simulink model "TRAS_pitch_model"  (Simulink 8.3)
settings: Solver=ode5  StartTime=0.0  StopTime=75  FixedStep=.01  RelTol=1e-3
PreLoadFcn:
  | load tras_char
undefined symbols (not defined in the file): control_p, force_p, rpm_p
settings Model: Creator=inteco  LastModifiedBy=inteco
settings DataIOCC: SignalLoggingName=sigsOut
settings OptimizationCC: ExpressionDepthLimit=2147483647
settings DebuggingCC: SaveWithParameterizedLinksMsg=none  SignalResolutionControl=TryResolveAllWithWarning  SolverPrmCheckMsg=none  MultiTaskDSMMsg=warning  MultiTaskCondExecSysMsg=none  FcnCallInpInsideContextMsg=UseLocalSettings  StrictBusMsg=None
settings HardwareCC: TargetUnknown=on
settings RTWCC: IncludeERTFirstTime=on

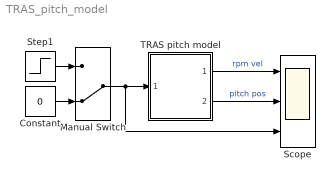
== system TRAS_pitch_model ==
  Constant : Constant  Value=0
  Manual Switch : ManualSwitch  CurrentSetting=0
  Scope : Scope  NumInputPorts=3
      settings: YMin=-250~-1.75~0  YMax=3250~1.75~1  MaxDataPoints=50000
  Step1 : Step  SampleTime=0
  TRAS pitch model : Subsystem
  wires:
  TRAS pitch model/2(pos_pm) -> Scope/2  "pitch pos"
  TRAS pitch model/1(rpm_p) -> Scope/1  "rpm vel"
  Step1/1 -> Manual Switch/1
  Constant/1 -> Manual Switch/2
  Manual Switch/1 -> TRAS pitch model/1(ctrl_p), Scope/3

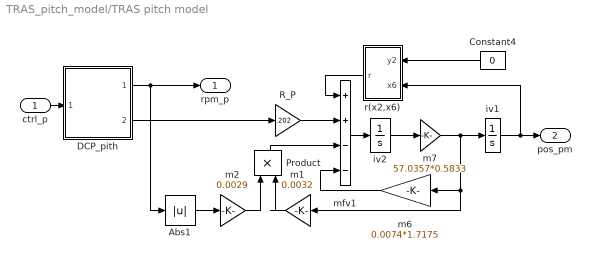
== system TRAS_pitch_model/TRAS pitch model ==
  ctrl_p : Inport
  Abs1 : Abs  SaturateOnIntegerOverflow=on
  Constant4 : Constant  Value=0
  DCP_pith : Subsystem
  Product : Product  SaturateOnIntegerOverflow=on  OutDataTypeStr=Inherit: Same as first input
  R_P : Gain  Gain=.202  OutDataTypeStr=Inherit: Same as input  ParamDataTypeStr=Inherit: Same as input
  iv1 : Integrator  LimitOutput=on  UpperSaturationLimit=pi/2  LowerSaturationLimit=-pi/2
  iv2 : Integrator  InitialCondition=-.1  UpperSaturationLimit=pi  LowerSaturationLimit=-pi
  m1 : Gain  Gain=0.0032  SaturateOnIntegerOverflow=on  OutDataTypeStr=Inherit: Same as input  ParamDataTypeStr=Inherit: Same as input
  m2 : Gain  Gain=0.0029  SaturateOnIntegerOverflow=on  OutDataTypeStr=Inherit: Same as input  ParamDataTypeStr=Inherit: Same as input
  m6 : Gain  Gain=0.0074*1.7175  OutDataTypeStr=Inherit: Same as input  ParamDataTypeStr=Inherit: Same as input
  m7 : Gain  Gain=57.0357*0.5833  SaturateOnIntegerOverflow=on  OutDataTypeStr=Inherit: Same as input  ParamDataTypeStr=Inherit: Same as input
  mfv1 : Sum  Inputs=++--  SaturateOnIntegerOverflow=on  InputSameDT=on  OutDataTypeStr=Inherit: Same as first input
  r(x2,x6) : Subsystem
  rpm_p : Outport
  pos_pm : Outport  Port=2
  wires:
  ctrl_p/1 -> DCP_pith/1(CTR_P)
  mfv1/1 -> iv2/1
  m2/1 -> Product/1
  m1/1 -> Product/2
  Constant4/1 -> r(x2,x6)/1(y2)
  r(x2,x6)/1(r) -> mfv1/1
  Product/1 -> mfv1/3
  Abs1/1 -> m2/1
  DCP_pith/1(RPM_P) -> rpm_p/1, Abs1/1
  m7/1 -> iv1/1, m6/1, m1/1
  iv2/1 -> m7/1
  m6/1 -> mfv1/4
  DCP_pith/2(FORCE_P) -> R_P/1
  R_P/1 -> mfv1/2
  iv1/1 -> pos_pm/1, r(x2,x6)/2(x6)

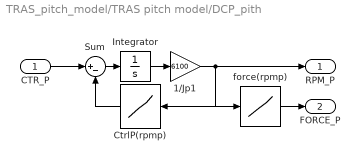
== system TRAS_pitch_model/TRAS pitch model/DCP_pith ==
  CTR_P : Inport
  1/Jp1 : Gain  Gain=6100  OutDataTypeStr=Inherit: Same as input  ParamDataTypeStr=Inherit: Same as input
  CtrlP(rpmp) : Lookup  InputValues=rpm_p  Table=control_p  SaturateOnIntegerOverflow=on
  Integrator : Integrator
  Sum : Sum  Inputs=|+-  SaturateOnIntegerOverflow=on  InputSameDT=on  OutDataTypeStr=Inherit: Same as first input
  force(rpmp) : Lookup  InputValues=rpm_p  Table=force_p  SaturateOnIntegerOverflow=on
  RPM_P : Outport
  FORCE_P : Outport  Port=2
  wires:
  force(rpmp)/1 -> FORCE_P/1
  CTR_P/1 -> Sum/1
  1/Jp1/1 -> RPM_P/1, force(rpmp)/1, CtrlP(rpmp)/1
  CtrlP(rpmp)/1 -> Sum/2
  Integrator/1 -> 1/Jp1/1
  Sum/1 -> Integrator/1

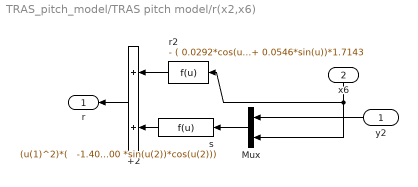
== system TRAS_pitch_model/TRAS pitch model/r(x2,x6) ==
  y2 : Inport
  x6 : Inport  Port=2
  +2 : Sum  SaturateOnIntegerOverflow=on  InputSameDT=on  OutDataTypeStr=Inherit: Same as first input
  Mux : Mux  Inputs=2
  r2 : Fcn  Expr=- ( 0.0292*cos(u)+ 0.0546*sin(u))*1.7143
  s : Fcn  Expr="(u(1)^2)*(   -1.40920355960000 *sin(u(2))*cos(u(2)))"
  r : Outport
  wires:
  +2/1 -> r/1
  y2/1 -> Mux/1
  x6/1 -> r2/1, Mux/2
  s/1 -> +2/2
  r2/1 -> +2/1
  Mux/1 -> s/1
